simulink model "meritve"  (R2020b)
settings: Solver=VariableStepAuto  StartTime=0.0  StopTime=15  RelTol=1e-3
libraries: simulink x2, PoKeysIOInterface x1
settings Model: Creator=64200047  LastModifiedBy=64200047

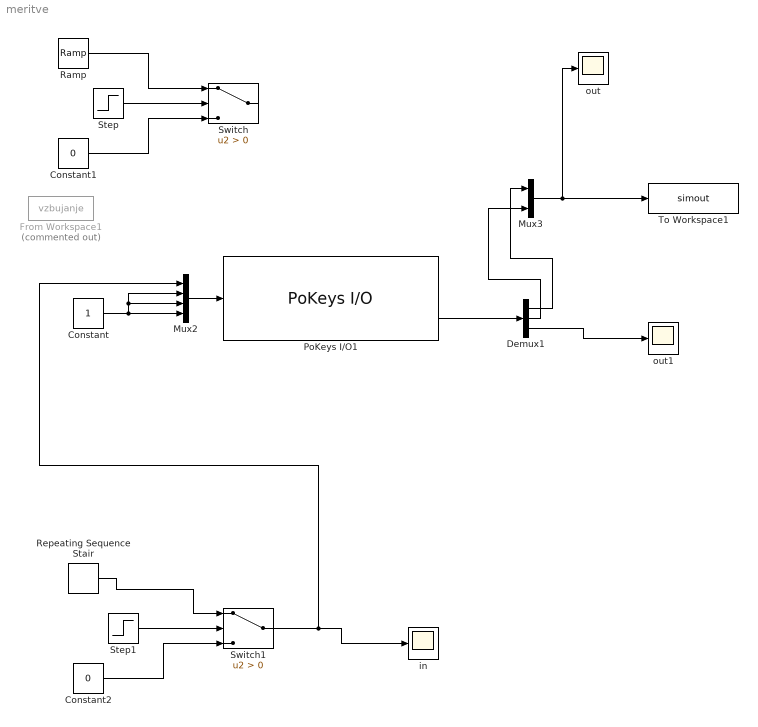
== system meritve ==
  Constant : Constant
  Constant1 : Constant  Value=0
  Constant2 : Constant  Value=0
  Demux1 : Demux  Outputs=3
  From Workspace1 : FromWorkspace  Commented=on  VariableName=vzbujanje
  Mux2 : Mux
  Mux3 : Mux  Inputs=2
  PoKeys I/O1 : PoKeysIOInterface/PoKeys I//O  MaxPowerLimit=100.0  IOTs=0.002  IOSerial=508
      settings: SourceProductName=PoKeys I/O interface
  Ramp : simulink/Sources/Ramp  slope=-2  start=0  InitialOutput=0
  Repeating Sequence Stair : simulink/Sources/Repeating Sequence Stair  OutValues=[8.5 -8.5].'  tsamp=0.5  OutMin=[]  OutMax=[]  OutDataTypeStr=double  OutputDataTypeScalingMode=double  OutDataType=fixdt(0,8)  ConRadixGroup=Best Precision: Vector-wise  OutScaling=2^-12
  Step : Step  Time=2  Before=2  After=0  SampleTime=0
  Step1 : Step  Before=2  After=0  SampleTime=0
  Switch : Switch  Criteria=u2 > Threshold
  Switch1 : Switch  Criteria=u2 > Threshold
  To Workspace1 : ToWorkspace  VariableName=simout  SaveFormat=Timeseries  SampleTime=-1
  in : Scope
  out : Scope
  out1 : Scope
  wires:
  Mux2/1 -> PoKeys I/O1/1
  PoKeys I/O1/2 -> Demux1/1
  Mux3/1 -> out/1, To Workspace1/1
  Demux1/1 -> Mux3/1
  Demux1/2 -> Mux3/2
  Demux1/3 -> out1/1
  Constant/1 -> Mux2/4, Mux2/3, Mux2/2
  Constant1/1 -> Switch/3
  Ramp/1 -> Switch/1
  Step/1 -> Switch/2
  Repeating Sequence Stair/1 -> Switch1/1
  Step1/1 -> Switch1/2
  Constant2/1 -> Switch1/3
  Switch1/1 -> Mux2/1, in/1
